simulink model "TP4_control_int_Haldane"  (R2024b)
settings: Solver=VariableStepAuto  StartTime=0.0  StopTime=10.0  FixedStep=0.  RelTol=1e-3
values from neighbouring files (symbols this model uses):
  e0 = mu_r*1.5    (= 0.12675)    [Main_entregable.m]
  states0 = [x0;s0]*1.5    [DatosModeloTP4.m]    (also in Main_entregable.m = [x0;s0;0;0]*1.5)
  v0 = 1    [DatosModeloTP4.m]
settings Model: Creator=tomii  LastModifiedBy=tomii

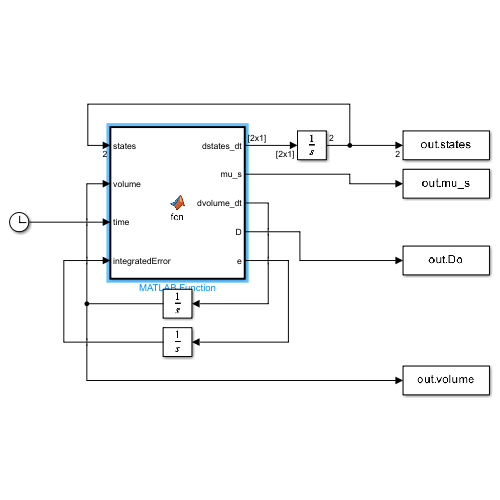
[thumbnail: Simulink's stored preview of the top-level diagram]
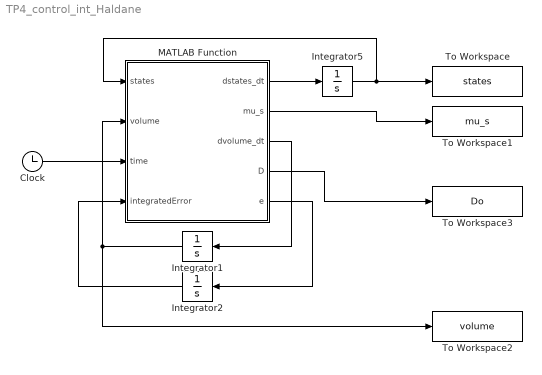
== system TP4_control_int_Haldane ==
  Clock : Clock
  Integrator1 : Integrator  InitialCondition=v0
  Integrator2 : Integrator  InitialCondition=e0
  Integrator5 : Integrator  InitialCondition=states0
  MATLAB Function : MATLAB Function  TreatAsAtomicUnit=on
  To Workspace : ToWorkspace  VariableName=states  SaveFormat=Timeseries  SampleTime=-1
  To Workspace1 : ToWorkspace  VariableName=mu_s  SaveFormat=Timeseries  SampleTime=-1
  To Workspace2 : ToWorkspace  VariableName=volume  SaveFormat=Timeseries  SampleTime=-1
  To Workspace3 : ToWorkspace  VariableName=Do  SaveFormat=Timeseries  SampleTime=-1
  wires:
  MATLAB Function/1(dstates_dt) -> Integrator5/1
  Integrator5/1 -> MATLAB Function/1(states), To Workspace/1
  MATLAB Function/2(mu_s) -> To Workspace1/1
  MATLAB Function/3(dvolume_dt) -> Integrator1/1
  Integrator1/1 -> MATLAB Function/2(volume), To Workspace2/1
  MATLAB Function/4(D) -> To Workspace3/1
  Clock/1 -> MATLAB Function/3(time)
  MATLAB Function/5(e) -> Integrator2/1
  Integrator2/1 -> MATLAB Function/4(integratedError)

== matlab function TP4_control_int_Haldane/MATLAB Function ==
  data: dstates_dt output; mu_s output; states input; volume input; time input; integratedError input; modelParameters parameter; dvolume_dt output; D output; e output
function [dstates_dt, mu_s, dvolume_dt, D, e] = fcn(states, volume, time, integratedError, modelParameters)   
    
    K=modelParameters.K;
    xi_in=modelParameters.xi_in;

    Ks=modelParameters.mu_model.Ks;
    Kis=modelParameters.mu_model.Kis;
    mu_max=modelParameters.mu_model.mu_max;
    mu_r=modelParameters.mu_r;
    s_r=modelParameters.s_r;
    x0=modelParameters.x0;
    s_in=modelParameters.s_in;
    kp=modelParameters.kp;
    ki=modelParameters.ki;
    
    x=states(1);
    s=states(2);

    mu_s=mu_max*(s/(s+Ks+s*s/Kis));
    rx=x*mu_s;

    e=(mu_r-mu_s);
    D=(1+kp*e+ki*integratedError)*(mu_r*Ks*x0*exp(time*mu_r))/(s_in-s_r);

    dstates_dt = K * rx + D*(xi_in-states);
    dvolume_dt = volume*D;

end
